simulink model "SpringMassDampingModel"  (R2021b)
settings: Solver=VariableStepAuto  StartTime=0.0  StopTime=1000  RelTol=1e-3
libraries: simulink x2
settings Model: Creator=Lenovo  LastModifiedBy=Lenovo

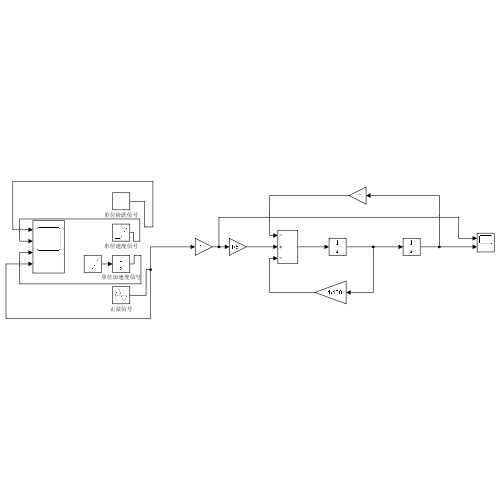
[thumbnail: Simulink's stored preview of the top-level diagram]
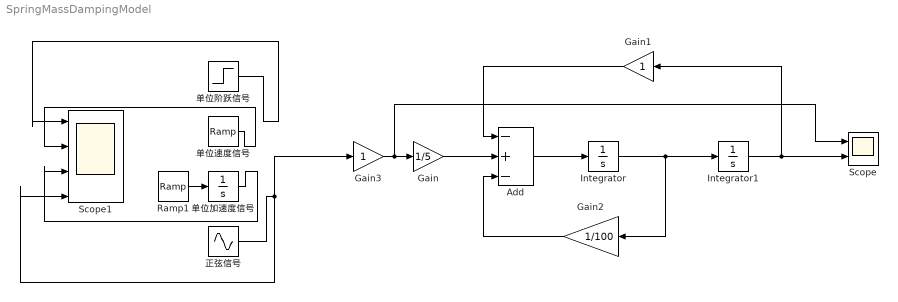
== system SpringMassDampingModel ==
  Add : Sum  Inputs=-+-
  Gain : Gain  Gain=1/5
  Gain1 : Gain
  Gain2 : Gain  Gain=1/100
  Gain3 : Gain
  Integrator : Integrator
  Integrator1 : Integrator
  Ramp1 : simulink/Sources/Ramp  slope=1  start=0  InitialOutput=0
  Scope : Scope  NumInputPorts=2
  Scope1 : Scope  NumInputPorts=4
  单位加速度信号 : Integrator
  单位速度信号 : simulink/Sources/Ramp  slope=1  start=0  InitialOutput=0
  单位阶跃信号 : Step  Time=0  SampleTime=0
  正弦信号 : Sin  SampleTime=0
  wires:
  Gain/1 -> Add/2
  Add/1 -> Integrator/1
  Gain1/1 -> Add/1
  Gain2/1 -> Add/3
  Integrator/1 -> Integrator1/1, Gain2/1
  Integrator1/1 -> Gain1/1, Scope/2
  单位速度信号/1 -> Scope1/2
  单位阶跃信号/1 -> Scope1/1
  正弦信号/1 -> Gain3/1, Scope1/4
  Ramp1/1 -> 单位加速度信号/1
  单位加速度信号/1 -> Scope1/3
  Gain3/1 -> Scope/1, Gain/1
